simulink model "sampleModel1792"  (R2023a)
settings: Solver=VariableStepAuto  StartTime=0.0  StopTime=10.0  RelTol=1e-3
libraries: hdlsllib x4, simulink x3
settings Model: Creator=user1  LastModifiedBy=user1

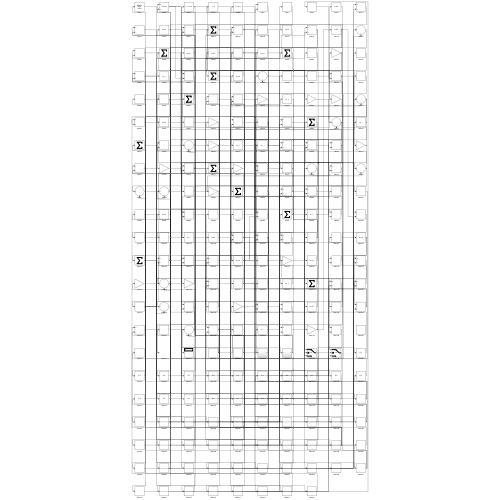
[thumbnail: Simulink's stored preview of the top-level diagram]
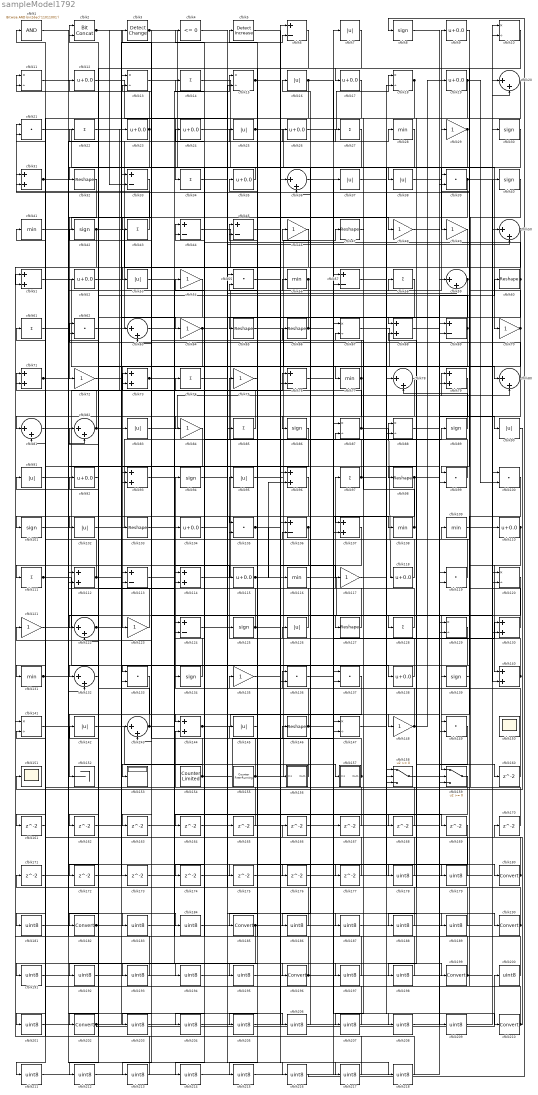
== system sampleModel1792 ==
  cfblk1 : simulink/Logic and Bit Operations/Bitwise Operator  logicop=AND  UseBitMask=on  BitMask=bin2dec('11011001')  BitMaskRealWorld=Stored Integer
      settings: LibrarySourceBlock=|
      | hdlsllib/Logic and Bit
      | Operations/Bitwise
      | Operator
  cfblk{10..11,13,15,18,67,87..88,120,129,141,147} (12 alike) : Product  Inputs=*/  RndMeth=Zero  SaturateOnIntegerOverflow=on
  cfblk{21,39,55,62,99..100,105,119,133,136..137,149} (12 alike) : DotProduct  OutDataTypeStr=Inherit: Inherit via internal rule
  cfblk{8,30,40,42,86,89,94,101,125,134,139} (11 alike) : Signum
  cfblk{7,16,25,37..38,53,83,90..91,95,102,126,142,145} (14 alike) : Abs  SaturateOnIntegerOverflow=off
  cfblk{32,47,60,65..66,98,103,127,146} (9 alike) : Reshape
  cfblk{9,12,17,19,23..24,26,35,52,92,104,110,115,118,138} (15 alike) : Bias  Bias=0.0  SaturateOnIntegerOverflow=off
  cfblk{6,33,44..45,57,69,76,106,113,124} (10 alike) : Sum  Inputs=+-
  cfblk{31,51,68,71,73,79,93,96,107,112,114,130,140,144} (14 alike) : Sum
  cfblk{28,41,56,77,108..109,116,131} (8 alike) : MinMax
  cfblk{14,22,27,34,43,58,61,74,85,97,111,128} (12 alike) : Sum  Inputs=+
  cfblk{29,46,48..49,54,64,70,72,75,84,117,121,123,135,148} (15 alike) : Gain
  cfblk{20,36,50,59,63,78,80..82,122,132,143} (12 alike) : Sum  Inputs=|++
  cfblk150 : Scope
      settings: Floating=on
  cfblk151 : Scope
  cfblk152 : Terminator
  cfblk153 : Display
  cfblk154 : hdlsllib/Sources/Counter Limited  uplimit=7  tsamp=-1
  cfblk155 : hdlsllib/Sources/Counter Free-Running  NumBits=16  tsamp=-1
  cfblk156 : Subsystem
      settings: LibrarySourceBlock=|
      | hdlsllib/Ports &
      | Subsystems/Subsystem
  cfblk157 : Subsystem
      settings: LibrarySourceBlock=|
      | hdlsllib/Ports &
      | Subsystems/Subsystem
  cfblk158 : Switch  SaturateOnIntegerOverflow=off  InputSameDT=off
  cfblk159 : Switch  SaturateOnIntegerOverflow=off  InputSameDT=off
  cfblk{160..177} (18 alike) : Delay  SampleTime=1
  cfblk{178..179,181,183..184,186..189,191..195,197..198,200..201,203..209,211..218} (33 alike) : DataTypeConversion  OutDataTypeStr=uint8  SaturateOnIntegerOverflow=off  RndMeth=Floor
  cfblk{180,182,185,190,196,199,202,210} (8 alike) : DataTypeConversion  SaturateOnIntegerOverflow=off  RndMeth=Floor
  cfblk2 : hdlsllib/Logic and Bit Operations/Bit Concat  numInputs=2
  cfblk3 : simulink/Logic and Bit Operations/Detect Change  vinit=0  OutDataTypeStr=boolean
      settings: LibrarySourceBlock=|
      | hdlsllib/Logic and Bit
      | Operations/Detect
      | Change
  cfblk4 : hdlsllib/Logic and Bit Operations/Compare To Zero  relop=<=  OutDataTypeStr=boolean
  cfblk5 : simulink/Logic and Bit Operations/Detect Increase  vinit=0.0  OutDataTypeStr=boolean
      settings: LibrarySourceBlock=|
      | hdlsllib/Logic and Bit
      | Operations/Detect
      | Increase
  wires:
  cfblk155/1 -> cfblk89/1, cfblk11/2
  cfblk32/1 -> cfblk72/1
  cfblk69/1 -> cfblk123/1, cfblk122/1, cfblk12/1
  cfblk121/1 -> cfblk23/1
  cfblk35/1 -> cfblk32/1
  cfblk64/1 -> cfblk83/1, cfblk59/2
  cfblk71/1 -> cfblk127/1, cfblk201/1
  cfblk26/1 -> cfblk18/1
  cfblk139/1 -> cfblk17/1
  cfblk40/1 -> cfblk146/1
  cfblk22/1 -> cfblk64/1
  cfblk133/1 -> cfblk152/1
  cfblk144/1 -> cfblk148/1, cfblk50/2
  cfblk88/1 -> cfblk90/1
  cfblk87/1 -> cfblk118/1, cfblk3/1
  cfblk80/1 -> cfblk62/1, cfblk211/1
  cfblk85/1 -> cfblk74/1
  cfblk17/1 -> cfblk102/1
  cfblk75/1 -> cfblk35/1
  cfblk18/1 -> cfblk34/1, cfblk111/1
  cfblk118/1 -> cfblk92/1
  cfblk90/1 -> cfblk151/1
  cfblk116/1 -> cfblk159/1
  cfblk157/1(Out1) -> cfblk71/1, cfblk66/1
  cfblk15/1 -> cfblk138/1, cfblk117/1
  cfblk117/1 -> cfblk78/1
  cfblk134/1 -> cfblk94/1
  cfblk37/1 -> cfblk180/1
  cfblk146/1 -> cfblk136/1, cfblk130/1, cfblk176/1
  cfblk102/1 -> cfblk88/1
  cfblk51/1 -> cfblk103/1
  cfblk114/1 -> cfblk9/1
  cfblk112/1 -> cfblk41/1, cfblk25/1
  cfblk95/1 -> cfblk47/1
  cfblk135/1 -> cfblk28/1
  cfblk81/1 -> cfblk76/1
  cfblk59/1 -> cfblk133/1, cfblk198/1
  cfblk29/1 -> cfblk144/1, cfblk194/1
  cfblk73/1 -> cfblk15/1, cfblk115/1
  cfblk96/1 -> cfblk101/1
  cfblk23/1 -> cfblk11/1, cfblk93/2
  cfblk147/1 -> cfblk210/1
  cfblk63/1 -> cfblk104/1
  cfblk57/1 -> cfblk190/1
  cfblk143/1 -> cfblk91/1, cfblk26/1
  cfblk14/1 -> cfblk49/1
  cfblk21/1 -> cfblk158/1
  cfblk56/1 -> cfblk93/1, cfblk84/1
  cfblk27/1 -> cfblk52/1
  cfblk131/1 -> cfblk114/2, cfblk56/1, cfblk27/1, cfblk179/1
  cfblk25/1 -> cfblk76/2, cfblk107/2
  cfblk154/1 -> cfblk87/1, cfblk42/1, cfblk153/1
  cfblk89/1 -> cfblk78/2
  cfblk3/1 -> cfblk88/2, cfblk43/1
  cfblk113/1 -> cfblk199/1
  cfblk138/1 -> cfblk95/1
  cfblk43/1 -> cfblk21/1
  cfblk92/1 -> cfblk22/1
  cfblk62/1 -> cfblk7/1
  cfblk105/1 -> cfblk79/1, cfblk116/1
  cfblk1/1 -> cfblk82/2
  cfblk50/1 -> cfblk81/1, cfblk128/1
  cfblk110/1 -> cfblk140/1, cfblk139/1
  cfblk16/1 -> cfblk108/1, cfblk63/2
  cfblk60/1 -> cfblk4/1, cfblk122/2
  cfblk65/1 -> cfblk110/1
  cfblk48/1 -> cfblk119/2
  cfblk123/1 -> cfblk2/1
  cfblk128/1 -> cfblk97/1
  cfblk145/1 -> cfblk185/1
  cfblk124/1 -> cfblk196/1
  cfblk106/1 -> cfblk133/2, cfblk161/1
  cfblk125/1 -> cfblk2/2, cfblk58/1, cfblk218/1
  cfblk142/1 -> cfblk157/1(In1)
  cfblk74/1 -> cfblk125/1
  cfblk19/1 -> cfblk98/1, cfblk100/2, cfblk172/1
  cfblk38/1 -> cfblk29/1
  cfblk99/1 -> cfblk54/1
  cfblk7/1 -> cfblk53/1
  cfblk67/1 -> cfblk79/2
  cfblk130/1 -> cfblk39/1
  cfblk34/1 -> cfblk69/2
  cfblk98/1 -> cfblk60/1, cfblk164/1
  cfblk137/1 -> cfblk182/1
  cfblk97/1 -> cfblk75/1, cfblk149/2
  cfblk109/1 -> cfblk140/2
  cfblk84/1 -> cfblk132/1
  cfblk108/1 -> cfblk67/2, cfblk87/2
  cfblk30/1 -> cfblk86/1
  cfblk42/1 -> cfblk51/2, cfblk96/1
  cfblk39/1 -> cfblk100/1, cfblk195/1
  cfblk49/1 -> cfblk131/1
  cfblk12/1 -> cfblk85/1
  cfblk126/1 -> cfblk45/1
  cfblk45/1 -> cfblk136/2
  cfblk41/1 -> cfblk48/1
  cfblk148/1 -> cfblk114/1, cfblk19/1
  cfblk24/1 -> cfblk70/1
  cfblk66/1 -> cfblk68/1, cfblk65/1, cfblk130/2
  cfblk52/1 -> cfblk80/1
  cfblk79/1 -> cfblk158/2
  cfblk6/1 -> cfblk105/1
  cfblk122/1 -> cfblk63/1, cfblk212/1
  cfblk8/1 -> cfblk39/2
  cfblk70/1 -> cfblk31/1, cfblk143/2
  cfblk111/1 -> cfblk158/3, cfblk175/1
  cfblk44/1 -> cfblk156/1(In1)
  cfblk9/1 -> cfblk99/1
  cfblk93/1 -> cfblk134/1
  cfblk119/1 -> cfblk44/1
  cfblk13/1 -> cfblk59/1
  cfblk10/1 -> cfblk202/1
  cfblk82/1 -> cfblk6/2, cfblk31/2
  cfblk100/1 -> cfblk149/1
  cfblk156/1(Out1) -> cfblk121/1
  cfblk115/1 -> cfblk36/1, cfblk96/2
  cfblk47/1 -> cfblk77/1
  cfblk2/1 -> cfblk33/1, cfblk33/2, cfblk38/1
  cfblk31/1 -> cfblk132/2, cfblk99/2
  cfblk127/1 -> cfblk73/1
  cfblk83/1 -> cfblk80/2
  cfblk77/1 -> cfblk13/2, cfblk204/1
  cfblk140/1 -> cfblk36/2, cfblk45/2
  cfblk58/1 -> cfblk107/1
  cfblk158/1 -> cfblk160/1
  cfblk160/1 -> cfblk105/2
  cfblk161/1 -> cfblk71/2
  cfblk33/1 -> cfblk162/1
  cfblk162/1 -> cfblk13/1
  cfblk54/1 -> cfblk163/1
  cfblk163/1 -> cfblk69/1
  cfblk164/1 -> cfblk15/2
  cfblk4/1 -> cfblk165/1
  cfblk165/1 -> cfblk82/1
  cfblk166/1 -> cfblk119/1
  cfblk76/1 -> cfblk167/1
  cfblk167/1 -> cfblk1/1
  cfblk103/1 -> cfblk168/1
  cfblk168/1 -> cfblk144/2
  cfblk36/1 -> cfblk169/1
  cfblk170/1 -> cfblk44/2
  cfblk171/1 -> cfblk112/2
  cfblk172/1 -> cfblk73/2
  cfblk72/1 -> cfblk173/1
  cfblk173/1 -> cfblk50/1
  cfblk107/1 -> cfblk174/1
  cfblk174/1 -> cfblk18/2
  cfblk175/1 -> cfblk159/3
  cfblk176/1 -> cfblk159/2
  cfblk53/1 -> cfblk177/1
  cfblk177/1 -> cfblk6/1
  cfblk5/1 -> cfblk178/1
  cfblk178/1 -> cfblk16/1
  cfblk179/1 -> cfblk5/1
  cfblk180/1 -> cfblk166/1, cfblk81/2
  cfblk86/1 -> cfblk181/1
  cfblk181/1 -> cfblk37/1
  cfblk182/1 -> cfblk143/1, cfblk67/1
  cfblk101/1 -> cfblk183/1
  cfblk183/1 -> cfblk137/1
  cfblk11/1 -> cfblk184/1
  cfblk184/1 -> cfblk137/2
  cfblk185/1 -> cfblk40/1, cfblk191/1
  cfblk28/1 -> cfblk186/1
  cfblk186/1 -> cfblk145/1
  cfblk55/1 -> cfblk187/1
  cfblk187/1 -> cfblk30/1
  cfblk149/1 -> cfblk188/1
  cfblk188/1 -> cfblk55/1
  cfblk94/1 -> cfblk189/1
  cfblk189/1 -> cfblk55/2
  cfblk190/1 -> cfblk68/2, cfblk61/1
  cfblk191/1 -> cfblk57/1
  cfblk132/1 -> cfblk192/1
  cfblk192/1 -> cfblk57/2
  cfblk120/1 -> cfblk193/1
  cfblk193/1 -> cfblk51/1
  cfblk194/1 -> cfblk120/1
  cfblk195/1 -> cfblk120/2
  cfblk196/1 -> cfblk112/1, cfblk21/2
  cfblk61/1 -> cfblk197/1
  cfblk197/1 -> cfblk124/1
  cfblk198/1 -> cfblk124/2
  cfblk199/1 -> cfblk24/1, cfblk14/1, cfblk135/1, cfblk126/1
  cfblk200/1 -> cfblk113/1
  cfblk201/1 -> cfblk113/2
  cfblk202/1 -> cfblk200/1, cfblk62/2
  cfblk78/1 -> cfblk203/1
  cfblk203/1 -> cfblk10/1
  cfblk204/1 -> cfblk10/2
  cfblk46/1 -> cfblk205/1
  cfblk205/1 -> cfblk106/1
  cfblk91/1 -> cfblk206/1
  cfblk206/1 -> cfblk46/1
  cfblk20/1 -> cfblk207/1
  cfblk207/1 -> cfblk106/2
  cfblk136/1 -> cfblk208/1
  cfblk208/1 -> cfblk20/1
  cfblk68/1 -> cfblk209/1
  cfblk209/1 -> cfblk20/2
  cfblk210/1 -> cfblk171/1, cfblk170/1, cfblk109/1
  cfblk211/1 -> cfblk147/1
  cfblk212/1 -> cfblk147/2
  cfblk129/1 -> cfblk213/1
  cfblk213/1 -> cfblk142/1
  cfblk159/1 -> cfblk214/1
  cfblk214/1 -> cfblk129/1
  cfblk169/1 -> cfblk215/1
  cfblk215/1 -> cfblk129/2
  cfblk141/1 -> cfblk216/1
  cfblk216/1 -> cfblk8/1
  cfblk104/1 -> cfblk217/1
  cfblk217/1 -> cfblk141/1
  cfblk218/1 -> cfblk141/2

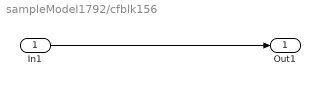
== system sampleModel1792/cfblk156 ==
  In1 : Inport
  Out1 : Outport
  wires:
  In1/1 -> Out1/1

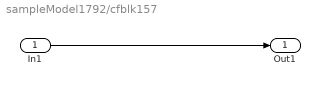
== system sampleModel1792/cfblk157 ==
  In1 : Inport
  Out1 : Outport
  wires:
  In1/1 -> Out1/1
